simulink model "record_realtime_model"  (R2024b)
settings: Solver=VariableStepAuto  StartTime=0.0  StopTime=10.0  RelTol=1e-3
libraries: dsparch4 x1, dspspect3 x1, dspnetwork x1
settings Model: Creator=roysi  LastModifiedBy=roysi

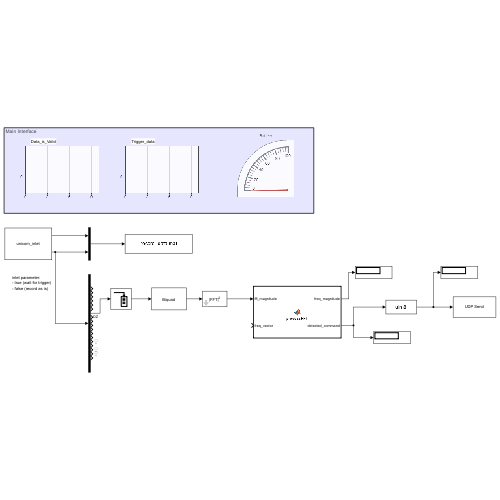
[thumbnail: Simulink's stored preview of the top-level diagram]
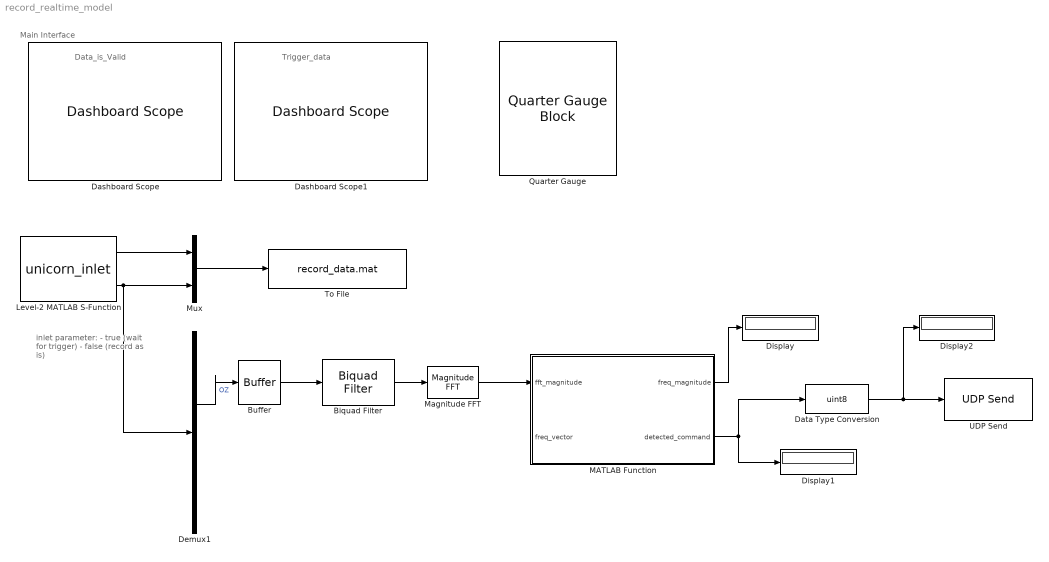
== system record_realtime_model ==
  note: Main Interface
  note: Trigger_data
  note: inlet parameter:
      | - true (wait for trigger)
      | - false (record as is)
  note: Data_is_Valid
  Biquad Filter : dsparch4/Biquad Filter  FilterSource=Dialog parameters  CoeffSource=Specify via dialog  FilterObject=BQF  IIRFiltStruct=Direct form II transposed  BiQuadCoeffs=[0.008826086668431, 0, -0.017652173336863, 1, 0, 0.008826086668431]  ScaleValues=1  IC=0  ICnum=0  ICden=0  a0Flag=Warning  optimizeScaleValues=on  ScaleValueMode=Specify via input port (g)  InputProcessing=Columns as channels (frame based)  roundingMode=Floor  overflowMode=off  scaleValueFracLength=14  denProdOutputFracLength=30  denAccumFracLength=30  secondMemoryFracLength=15
  Buffer : Buffer  OutputFrames=off
  Dashboard Scope : DashboardScope  Ymin=-1  Ymax=2
  Dashboard Scope1 : DashboardScope  Ymin=-1  Ymax=2
  Data Type Conversion : DataTypeConversion  OutDataTypeStr=uint8  RndMeth=Nearest  SaturateOnIntegerOverflow=off
  Demux1 : Demux  Outputs=18
  Display : Display
  Display1 : Display
  Display2 : Display
  Level-2 MATLAB S-Function : M-S-Function  FunctionName=unicorn_inlet  Parameters=false
  MATLAB Function : MATLAB Function  TreatAsAtomicUnit=on
  Magnitude FFT : dspspect3/Magnitude FFT  mag_or_magsq=Magnitude squared  FFTImplementation=Auto  fftLenInherit=off  fftsize=256  WrapInput=on
      settings: LibrarySourceBlock=|
      | dspxfrm3/Magnitude
      | FFT
  Mux : Mux  Inputs=2
  Quarter Gauge : QuarterGaugeBlock
  To File : ToFile  Filename=record_data.mat  MatrixName=y
  UDP Send : dspnetwork/UDP Send  remoteURL='127.0.0.1'  remotePort=25000  localURL='0.0.0.0'  localPortSource=Automatically determine  localPort=-1  sendBufferSize=8192  sampletime=-1  blockPlatform=[]  separateLengthPort=0
      settings: LibrarySourceBlock=dspsnks4/UDP Send
  wires:
  Mux/1 -> To File/1
  Level-2 MATLAB S-Function/2 -> Demux1/1, Mux/2
  Level-2 MATLAB S-Function/1 -> Mux/1
  Demux1/7 -> Buffer/1  "OZ"
  Data Type Conversion/1 -> Display2/1, UDP Send/1
  MATLAB Function/1(freq_magnitude) -> Display/1
  Buffer/1 -> Biquad Filter/1
  Magnitude FFT/1 -> MATLAB Function/1(fft_magnitude)
  Biquad Filter/1 -> Magnitude FFT/1
  MATLAB Function/2(detected_command) -> Data Type Conversion/1, Display1/1

== matlab function record_realtime_model/MATLAB Function ==
  data: fft_magnitude input; freq_magnitude output; freq_vector input; detected_command output
function [freq_magnitude, detected_command] = processFFT(fft_magnitude, freq_vector)
    % Define frequency bands (corresponding to stimulus frequencies)
    stimulus_frequencies = [9, 13, 15, 17]; % Hz
    tolerance = 0.5; % Allowable frequency error margin

    % Initialize outputs
    detected_command = 0; % Default if no match is found
    freq_magnitude = 0; % Default magnitude value
    
    % Find the frequency bin with the maximum magnitude
    [max_magnitude, max_idx] = max(fft_magnitude);
    detected_freq = freq_vector(max_idx); % Corresponding frequency value

    % Check which predefined band the detected frequency belongs to
    for i = 1:length(stimulus_frequencies)
        if abs(detected_freq - stimulus_frequencies(i)) < tolerance
            detected_command = i; % 1 for 9Hz, 2 for 13Hz, etc.
            freq_magnitude = max_magnitude; % Assign the max magnitude
            return;
        end
    end
end
